simulink model "sf_mandelbrot_fixpt"  (Simulink 6.0)
settings: Solver=FixedStepDiscrete  SolverMode=SingleTasking  StartTime=0.0  StopTime=inf  FixedStep=0.0005  RelTol=1e-3
CloseFcn:
  | sf_mandel_gui('close');
settings Model: CovMetricSettings=dcmtr  Creator=The MathWorks Inc.  LastModifiedBy=batserve  ExtModeAutoUpdateStatusClock=off
settings DataIOCC: SaveOutput=off  SaveTime=off
settings OptimizationCC: BooleanDataType=off  InlineInvariantSignals=off
settings DebuggingCC: CheckExecutionContextPreStartOutputMsg=on  CheckExecutionContextRuntimeOutputMsg=on  SolverPrmCheckMsg=none
settings HardwareCC: TargetUnknown=on

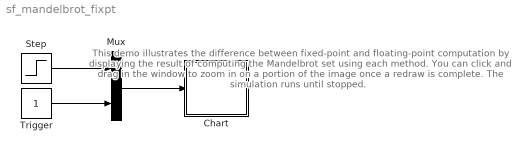
== system sf_mandelbrot_fixpt ==
  note: This demo illustrates the difference between
      | fixed-point and floating-point computation by
      | displaying the result of computing the
      | Mandelbrot set using each method.
      |
      | You can click and drag in the window to zoom
      | in on a portion of the image once a redraw is
      | complete. The simulation runs until stopped.
  Chart : Stateflow chart  Orientation=down  TreatAsAtomicUnit=on  PropExecContextAcrossSSBoundary=on
  Mux : Mux  Inputs=2
  Step : Step  Time=0.1  SampleTime=0  ZeroCross=off
  Trigger : Constant
  wires:
  Trigger/1 -> Mux/2
  Step/1 -> Mux/1
  Mux/1 -> Chart/Trigger

== stateflow chart Chart ==
  state i = mandel_fix(a0,b0) [function]
    (default) -> (junction 6) : { i = 0;
        |  r2 = 0;
        |  local_colors = colors; }
    (junction 6) -> (junction 7) : {
        | bn = 2 * an * bn + b0;
        | an = r2 + a0;
        | r2 = an * an - bn * bn;
        | }
    (junction 11) -> (junction 8) : {
        | i++;
        | }
    (junction 8) -> (junction 6)
    (junction 7) -> (junction 9)
    (junction 7) -> (junction 11) : [ r2 < 4 && i < local_colors ]
  state Wait
    entry:ml.sf_mandel_gui("enter_wait");
  state i = mandel_double(a0,b0) [function]
    (junction 20) -> (junction 22) : [ r2 < 4 && i < local_colors ]
    (junction 20) -> (junction 18)
    (junction 19) -> (junction 21)
    (junction 22) -> (junction 19) : {
        | i++;
        | }
    (junction 21) -> (junction 20) : {
        | bn = 2 * an * bn + b0;
        | an = r2 + a0;
        | r2 = an * an - bn * bn;
        | }
    (default) -> (junction 21) : { i = 0;
        |  r2 = 0;
        |  local_colors = colors; }
  (junction 15) -> Wait : { ml.toc() }
  (junction 17) -> (junction 10) : {
      | fix_line[j]  = mandel_fix(x,y0);
      | dbl_line[j] = mandel_double(x,y0);
      | }
  (junction 10) -> (junction 12)
  (junction 12) -> (junction 13) : {
      | j++;
      | x += deltax;
      | }
  (default) -> (junction 14) : Start {
      | 1
      | ml.sf_mandel_gui();
      | }
  (junction 23) -> (junction 15)
  (junction 15) -> (junction 16) : [ i <= pix_h ]
  (junction 16) -> (junction 17) : {
      | j = 1;
      | x = real_left;
      | }
  (junction 13) -> (junction 17) : [ j <= pix_w]
  (junction 13) -> (junction 15) : {
      | ml.sf_mandel_gui(i,dbl_line,fix_line);
      | ml.sf_mandel_gui("update");
      | i++;
      | y0 -= deltay;
      | }
  (junction 14) -> (junction 23) : {
      | ml.sf_mandel_gui("exit_wait");
      | colors = ml.sf_mandel_gui("colors");
      |
      | pix_w = ml.sf_mandel_gui("pixel width");
      | pix_h  = ml.sf_mandel_gui("pixel height");
      |
      | real_left = ml.sf_mandel_gui("real left");
      | real_top = ml.sf_mandel_gui("real top");
      | real_w   = ml.sf_mandel_gui("real width");
      | real_h   = ml.sf_mandel_gui("real height");
      |
      | deltax = real_w / pix_w;
      | deltay = real_h / pix_h;
      |
      | i=1;
      | y0 = real_top;
      | ml.tic();
      | }
  Wait -> (junction 14) : Redraw
  data: a0 function_input fixpt; b0 function_input fixpt; an temporary fixpt; bn temporary fixpt; bt temporary fixpt; i function_output int32; r2 temporary fixpt; local_colors temporary int32; a0 function_input double; b0 function_input double; an temporary double; bn temporary double; bt temporary double; i function_output int32; local_colors temporary int32; r2 temporary double; real_left local double; real_w local double; pix_w local double; deltax local double; deltay local double; i local int32; y0 local double; j local int32; x local double; real_top local double; real_h local double; pix_h local double; colors local double; dbl_c local double; fix_c local double; fix_line local double size=1024; dbl_line local double size=1024
  events: Start input EITHER_EDGE_EVENT; Redraw input EITHER_EDGE_EVENT
